simulink model "thesis"  (R2021b)
settings: Solver=VariableStepAuto  StartTime=0.0  StopTime=inf  RelTol=1e-3
values from neighbouring files (symbols this model uses):
  f = 7489    [traj.m]
libraries: instrumentlib x2
settings Model: Creator=alekh  LastModifiedBy=alekh

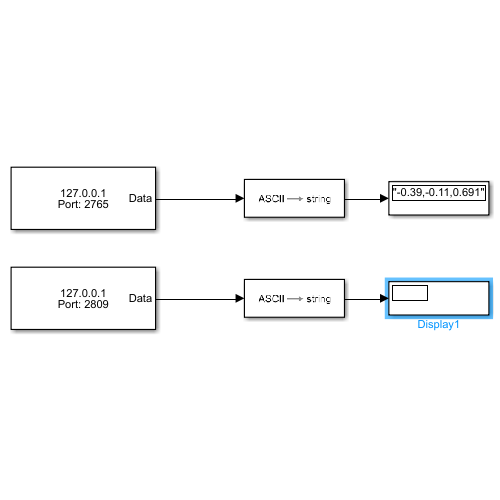
[thumbnail: Simulink's stored preview of the top-level diagram]
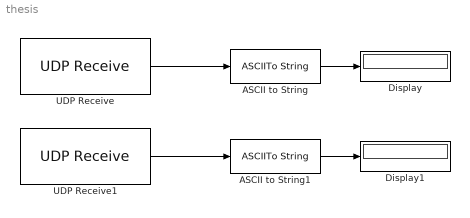
== system thesis ==
  ASCII to String : ASCIIToString
  ASCII to String1 : ASCIIToString
  Display : Display
  Display1 : Display
  UDP Receive : instrumentlib/UDP Receive  Host=localhost  Port=9090  LocalPort=2765  EnablePortSharing=off  GetLatestData=off  DataSize="[17   1]"  DataType=uint8  ASCIIFormatting=%f,  Terminator=LF  ByteOrder=BigEndian  EnableBlockingMode=on  Timeout=10  SampleTime=0.01  LocalAddress=127.0.0.1
  UDP Receive1 : instrumentlib/UDP Receive  Host=localhost  Port=9090  LocalPort=2809  EnablePortSharing=off  GetLatestData=off  DataSize="[5  1]"  DataType=uint8  ASCIIFormatting=%f,  Terminator=LF  ByteOrder=BigEndian  EnableBlockingMode=on  Timeout=10  SampleTime=0.01  LocalAddress=127.0.0.1
  wires:
  UDP Receive/1 -> ASCII to String/1
  ASCII to String/1 -> Display/1
  UDP Receive1/1 -> ASCII to String1/1
  ASCII to String1/1 -> Display1/1
